simulink model "gm_smartCart3111"  (R2016a)
settings: Solver=FixedStepDiscrete  StartTime=0.0  StopTime=inf  FixedStep=1  RelTol=1e-3
libraries: simulink x92, hdlsllib x50
(part 1 of 3)
settings Model: Creator=Admin  LastModifiedBy=Admin
settings OptimizationCC: BlockReduction=off  ConditionallyExecuteInputs=off  DefaultParameterBehavior=Inlined
settings DebuggingCC: AlgebraicLoopMsg=error  InheritedTsInSrcMsg=none  MultiTaskCondExecSysMsg=warning  MultiTaskRateTransMsg=warning
settings HardwareCC: ProdBitPerPointer=32  ProdLargestAtomicFloat=None  ProdIntDivRoundTo=Undefined  ProdEndianess=Unspecified  ProdWordSize=32  ProdHWDeviceType=ASIC/FPGA->ASIC/FPGA  ProdEqTarget=off

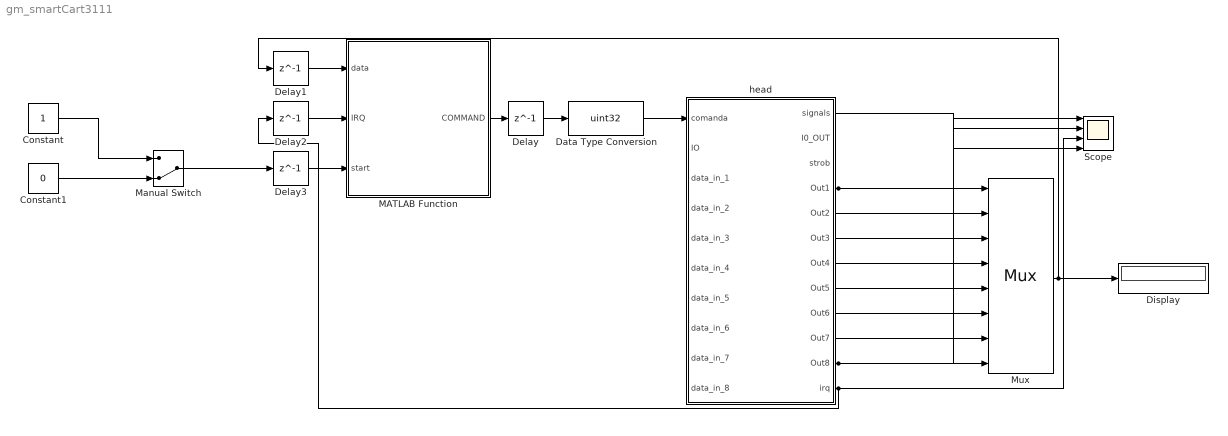
== system gm_smartCart3111 ==
  Constant : Constant  OutDataTypeStr=uint8
  Constant1 : Constant  Value=0  OutDataTypeStr=uint8
  Data Type Conversion : DataTypeConversion  OutDataTypeStr=uint32
  Delay{,1..3} (4 alike) : Delay  DelayLength=1  InitialCondition=0
  Display : Display
  MATLAB Function : MATLAB Function  TreatAsAtomicUnit=on
  Manual Switch : ManualSwitch  CurrentSetting=0
  Mux : Mux  Inputs=8
  Scope : Scope  NumInputPorts=4
  head : Subsystem  TreatAsAtomicUnit=on
  wires:
  Manual Switch/1 -> Delay3/1
  Delay3/1 -> MATLAB Function/3(start)
  Delay2/1 -> MATLAB Function/2(IRQ)
  Delay1/1 -> MATLAB Function/1(data)
  MATLAB Function/1(COMMAND) -> Delay/1
  Delay/1 -> Data Type Conversion/1
  head/1(signals) -> Scope/4
  head/11(Out8) -> Mux/8, Scope/2
  Data Type Conversion/1 -> head/1(comanda)
  Mux/1 -> Display/1, Delay1/1
  head/10(Out7) -> Mux/7
  head/9(Out6) -> Mux/6
  head/8(Out5) -> Mux/5
  head/7(Out4) -> Mux/4
  head/6(Out3) -> Mux/3
  head/5(Out2) -> Mux/2
  head/4(Out1) -> Mux/1, Scope/1
  head/12(irq) -> Scope/3, Delay2/1
  Constant1/1 -> Manual Switch/2
  Constant/1 -> Manual Switch/1

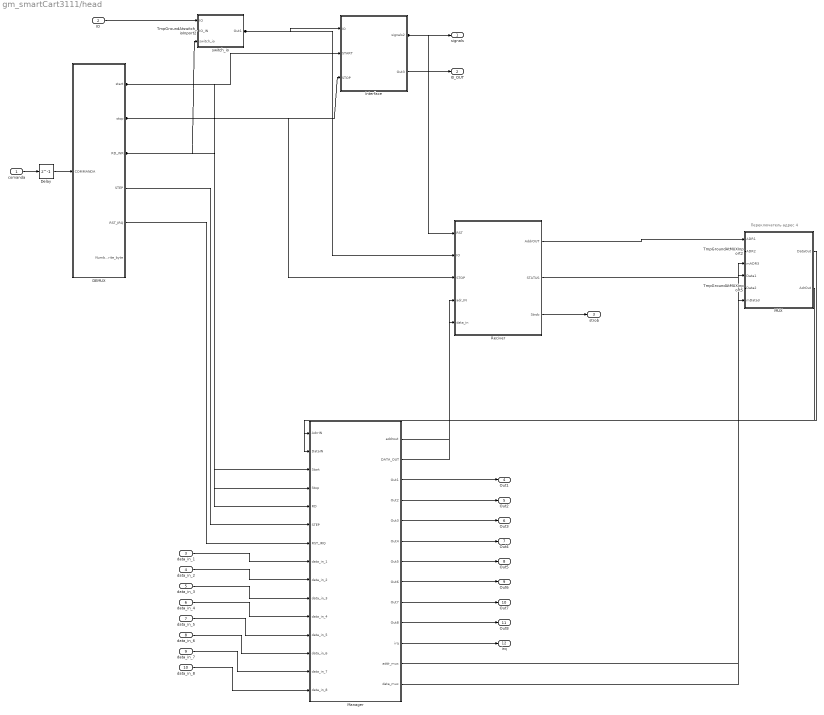
== system gm_smartCart3111/head ==
  note: Переключатель адрес 4
  comanda : Inport  OutDataTypeStr=uint32  SampleTime=1
  IO : Inport  Port=2  OutDataTypeStr=boolean
  data_in_1 : Inport  Port=3  OutDataTypeStr=uint32
  data_in_2 : Inport  Port=4  OutDataTypeStr=uint32
  data_in_3 : Inport  Port=5  OutDataTypeStr=uint32
  data_in_4 : Inport  Port=6  OutDataTypeStr=uint32
  data_in_5 : Inport  Port=7  OutDataTypeStr=uint32
  data_in_6 : Inport  Port=8  OutDataTypeStr=uint32
  data_in_7 : Inport  Port=9  OutDataTypeStr=uint32
  data_in_8 : Inport  Port=10  OutDataTypeStr=uint32
  DEMUX : Subsystem
  Delay : Delay  DelayLength=1  InitialCondition=0
  Interface : Subsystem
  MUX : Subsystem
  Manager : Subsystem
  Reciver : Subsystem
  TmpGroundAtMUXInport2 : Ground  DisableCoverage=on
  TmpGroundAtMUXInport5 : Ground  DisableCoverage=on
  TmpGroundAtswitch_ioInport2 : Ground  DisableCoverage=on
  switch_io : Subsystem
  signals : Outport  OutDataTypeStr=fixdt(1,4,0)
  I0_OUT : Outport  Port=2  OutDataTypeStr=boolean
  strob : Outport  Port=3  OutDataTypeStr=boolean
  Out1 : Outport  Port=4  OutDataTypeStr=uint8
  Out2 : Outport  Port=5  OutDataTypeStr=uint8
  Out3 : Outport  Port=6  OutDataTypeStr=uint8
  Out4 : Outport  Port=7  OutDataTypeStr=uint8
  Out5 : Outport  Port=8  OutDataTypeStr=uint8
  Out6 : Outport  Port=9  OutDataTypeStr=uint8
  Out7 : Outport  Port=10  OutDataTypeStr=uint8
  Out8 : Outport  Port=11  OutDataTypeStr=uint8
  irq : Outport  Port=12  OutDataTypeStr=boolean
  wires:
  comanda/1 -> Delay/1
  IO/1 -> switch_io/1(IO)
  data_in_1/1 -> Manager/8(data_in_1)
  data_in_2/1 -> Manager/9(data_in_2)
  data_in_3/1 -> Manager/10(data_in_3)
  data_in_4/1 -> Manager/11(data_in_4)
  data_in_5/1 -> Manager/12(data_in_5)
  data_in_6/1 -> Manager/13(data_in_6)
  data_in_7/1 -> Manager/14(data_in_7)
  data_in_8/1 -> Manager/15(data_in_8)
  DEMUX/1(start) -> Interface/2(START), Manager/3(Start)
  DEMUX/2(stop) -> Interface/3(STOP), Reciver/3(STOP), Manager/4(Stop)
  DEMUX/3(RD_WR) -> switch_io/3(switch_io), Manager/5(RD)
  DEMUX/4(STEP) -> Manager/6(STEP)
  DEMUX/5(RST_IRQ) -> Manager/7(RST_IRQ)
  Delay/1 -> DEMUX/1(COMMANDA)
  Interface/1(signals2) -> Reciver/1(RST), signals/1
  Interface/2(Out3) -> I0_OUT/1
  MUX/1(DataOut) -> Manager/2(DataIN)
  MUX/2(AdrOut) -> Manager/1(AdrrIN)
  Manager/1(addrout) -> Reciver/4(adr_IN)
  Manager/2(DATA_OUT) -> Reciver/5(data_in)
  Manager/3(Out1) -> Out1/1
  Manager/4(Out2) -> Out2/1
  Manager/5(Out3) -> Out3/1
  Manager/6(Out4) -> Out4/1
  Manager/7(Out5) -> Out5/1
  Manager/8(Out6) -> Out6/1
  Manager/9(Out7) -> Out7/1
  Manager/10(Out8) -> Out8/1
  Manager/11(irq) -> irq/1
  Manager/12(addr_mux) -> MUX/3(mADR3)
  Manager/13(data_mux) -> MUX/6(mData3)
  Reciver/1(AddrOUT) -> MUX/1(ADR1)
  Reciver/2(STATUS) -> MUX/4(Data1)
  Reciver/3(Strob) -> strob/1
  TmpGroundAtMUXInport2/1 -> MUX/2(ADR2)
  TmpGroundAtMUXInport5/1 -> MUX/5(Data2)
  TmpGroundAtswitch_ioInport2/1 -> switch_io/2(IO_IN)
  switch_io/1(Out1) -> Interface/1(IO), Reciver/2(IO)

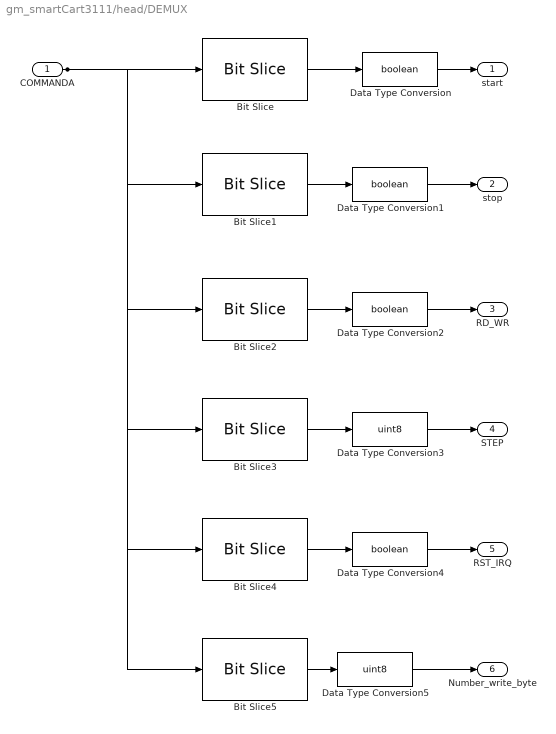
== system gm_smartCart3111/head/DEMUX ==
  COMMANDA : Inport  OutDataTypeStr=uint32  SampleTime=1
  Bit Slice : hdlsllib/HDL Operations/Bit Slice  lidx=0  ridx=0
  Bit Slice1 : hdlsllib/HDL Operations/Bit Slice  lidx=1  ridx=1
  Bit Slice2 : hdlsllib/HDL Operations/Bit Slice  lidx=2  ridx=2
  Bit Slice3 : hdlsllib/HDL Operations/Bit Slice  lidx=11  ridx=3
  Bit Slice4 : hdlsllib/HDL Operations/Bit Slice  lidx=12  ridx=12
  Bit Slice5 : hdlsllib/HDL Operations/Bit Slice  lidx=15  ridx=13
  Data Type Conversion{,1..2,4} (4 alike) : DataTypeConversion  OutDataTypeStr=boolean
  Data Type Conversion3 : DataTypeConversion  OutDataTypeStr=uint8
  Data Type Conversion5 : DataTypeConversion  OutDataTypeStr=uint8
  start : Outport
  stop : Outport  Port=2
  RD_WR : Outport  Port=3
  STEP : Outport  Port=4  OutDataTypeStr=uint8
  RST_IRQ : Outport  Port=5
  Number_write_byte : Outport  Port=6  OutDataTypeStr=uint8
  wires:
  COMMANDA/1 -> Bit Slice5/1, Bit Slice4/1, Bit Slice3/1, Bit Slice2/1, Bit Slice1/1, Bit Slice/1
  Bit Slice/1 -> Data Type Conversion/1
  Bit Slice1/1 -> Data Type Conversion1/1
  Bit Slice2/1 -> Data Type Conversion2/1
  Bit Slice3/1 -> Data Type Conversion3/1
  Bit Slice4/1 -> Data Type Conversion4/1
  Bit Slice5/1 -> Data Type Conversion5/1
  Data Type Conversion/1 -> start/1
  Data Type Conversion1/1 -> stop/1
  Data Type Conversion2/1 -> RD_WR/1
  Data Type Conversion3/1 -> STEP/1
  Data Type Conversion4/1 -> RST_IRQ/1
  Data Type Conversion5/1 -> Number_write_byte/1

== system gm_smartCart3111/head/Interface ==
  IO : Inport  OutDataTypeStr=boolean
  START : Inport  Port=2  OutDataTypeStr=boolean  SampleTime=1
  STOP : Inport  Port=3  OutDataTypeStr=boolean  SampleTime=1
  ColdStart : Subsystem
  ColdStop2 : Subsystem
  Head2 : Subsystem
  MUX2 : Subsystem
  Swith_signal2 : Subsystem
  signals2 : Outport  OutDataTypeStr=fixdt(1,4,0)  InitialOutput=0
  Out3 : Outport  Port=2  OutDataTypeStr=boolean  InitialOutput=0
  wires:
  IO/1 -> Out3/1, ColdStart/1(Reqest)
  START/1 -> Head2/3(START)
  STOP/1 -> Head2/4(STOP)
  ColdStart/1(DataOUT) -> MUX2/5(DAT_ST1)
  ColdStart/2(Signal) -> MUX2/2(DATA_0)
  ColdStart/3(ADR_OUT) -> MUX2/4(ADR_ST)
  ColdStop2/1(DataOUT) -> MUX2/7(DAT_STOP)
  ColdStop2/2(Signal) -> MUX2/3(DATA_1)
  ColdStop2/3(ADR_OUT) -> MUX2/6(ADR_STOP)
  Head2/1(AdrOut) -> Swith_signal2/1(Adr), ColdStart/2(Addr), ColdStop2/1(Addr)
  Head2/2(DataOut) -> Swith_signal2/2(Data), ColdStart/3(Data), ColdStop2/2(Data)
  MUX2/1(Signals) -> signals2/1
  MUX2/2(ADR_OUT) -> Head2/1(ADR_IN)
  MUX2/3(DATA_OUT1) -> Head2/2(DataIN)
  Swith_signal2/1(OutAddr) -> MUX2/1(ADR)

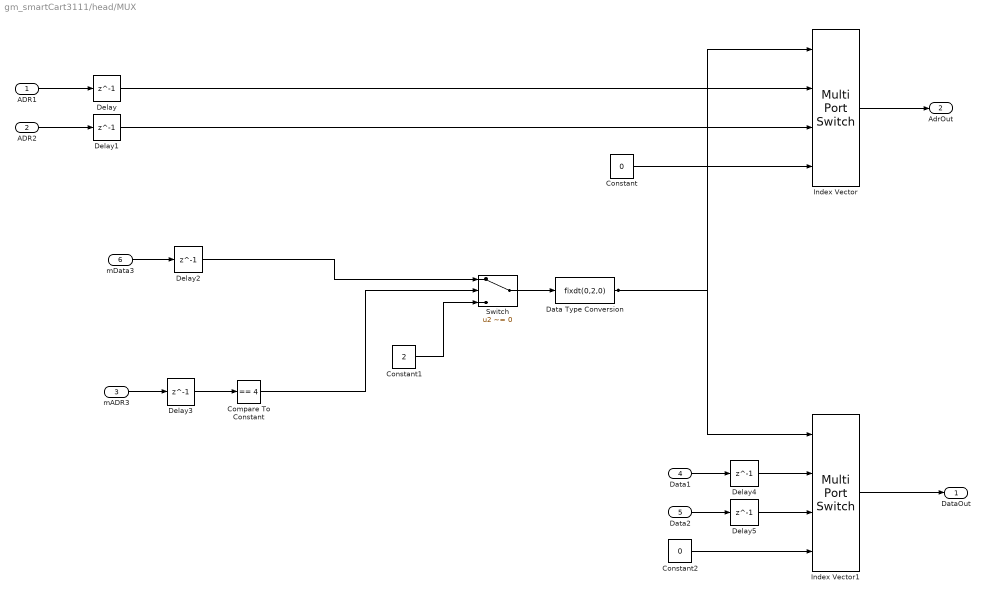
== system gm_smartCart3111/head/MUX ==
  ADR1 : Inport  OutDataTypeStr=uint8  SampleTime=1
  ADR2 : Inport  Port=2  OutDataTypeStr=uint8
  mADR3 : Inport  Port=3  OutDataTypeStr=uint8  SampleTime=1
  Data1 : Inport  Port=4  OutDataTypeStr=uint32  SampleTime=1
  Data2 : Inport  Port=5  OutDataTypeStr=uint32
  mData3 : Inport  Port=6  OutDataTypeStr=uint32  SampleTime=1
  Compare To Constant : simulink/Logic and Bit Operations/Compare To Constant  relop===  const=4  OutDataTypeStr=boolean
  Constant : Constant  Value=0  OutDataTypeStr=uint8
  Constant1 : Constant  Value=2  OutDataTypeStr=uint32
  Constant2 : Constant  Value=0  OutDataTypeStr=uint32
  Data Type Conversion : DataTypeConversion  OutDataTypeStr=fixdt(0,2,0)
  Delay{,1..5} (6 alike) : Delay  DelayLength=1  InitialCondition=0
  Index Vector : MultiPortSwitch  DataPortOrder=Zero-based contiguous  zeroidx=on
  Index Vector1 : MultiPortSwitch  DataPortOrder=Zero-based contiguous  zeroidx=on
  Switch : Switch  Criteria=u2 ~= 0
  DataOut : Outport  OutDataTypeStr=uint32
  AdrOut : Outport  Port=2  OutDataTypeStr=uint8
  wires:
  ADR1/1 -> Delay/1
  ADR2/1 -> Delay1/1
  mADR3/1 -> Delay3/1
  Data1/1 -> Delay4/1
  Data2/1 -> Delay5/1
  mData3/1 -> Delay2/1
  Compare To Constant/1 -> Switch/2
  Constant/1 -> Index Vector/4
  Constant1/1 -> Switch/3
  Constant2/1 -> Index Vector1/4
  Data Type Conversion/1 -> Index Vector1/1, Index Vector/1
  Delay/1 -> Index Vector/2
  Delay1/1 -> Index Vector/3
  Delay2/1 -> Switch/1
  Delay3/1 -> Compare To Constant/1
  Delay4/1 -> Index Vector1/2
  Delay5/1 -> Index Vector1/3
  Index Vector/1 -> AdrOut/1
  Index Vector1/1 -> DataOut/1
  Switch/1 -> Data Type Conversion/1

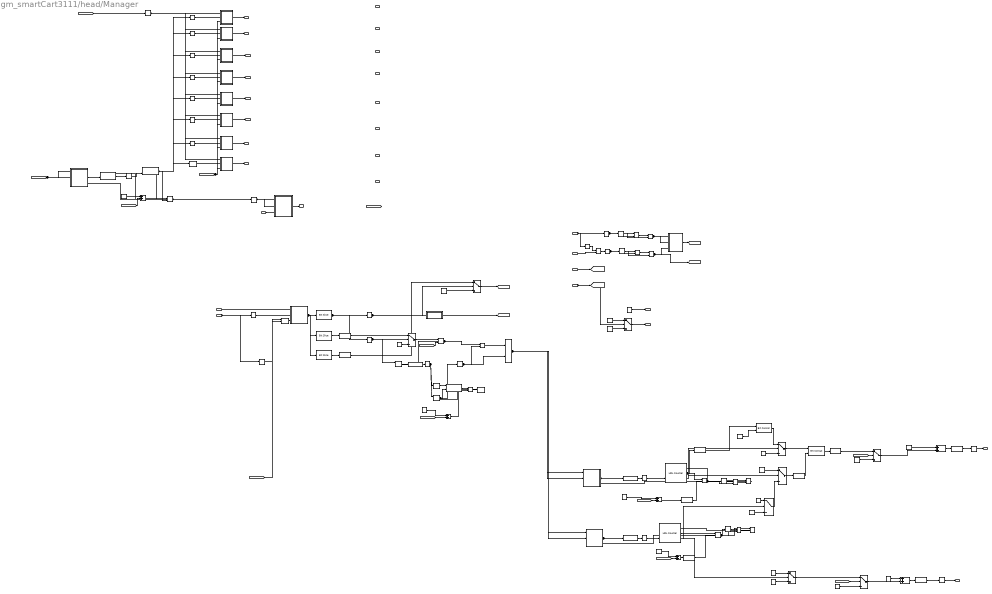
== system gm_smartCart3111/head/Manager ==
  note: Схема управления приёмника
  note: Схема включения и выключения
  note: Схема синхр
  note: Схема декодирования команд
  note: Декодер команд
  AdrrIN : Inport  OutDataTypeStr=uint8  SampleTime=1
  DataIN : Inport  Port=2  OutDataTypeStr=uint32  SampleTime=1
  Start : Inport  Port=3  OutDataTypeStr=boolean  SampleTime=1
  Stop : Inport  Port=4  OutDataTypeStr=boolean  SampleTime=1
  RD : Inport  Port=5  OutDataTypeStr=boolean  SampleTime=1
  STEP : Inport  Port=6  OutDataTypeStr=uint8  SampleTime=1
  RST_IRQ : Inport  Port=7  OutDataTypeStr=boolean  SampleTime=1
  data_in_1 : Inport  Port=8  OutDataTypeStr=uint32
  data_in_2 : Inport  Port=9  OutDataTypeStr=uint32
  data_in_3 : Inport  Port=10  OutDataTypeStr=uint32
  data_in_4 : Inport  Port=11  OutDataTypeStr=uint32
  data_in_5 : Inport  Port=12  OutDataTypeStr=uint32
  data_in_6 : Inport  Port=13  OutDataTypeStr=uint32
  data_in_7 : Inport  Port=14  OutDataTypeStr=uint32
  data_in_8 : Inport  Port=15  OutDataTypeStr=uint32
  Add{,1..5} (6 alike) : Sum
  Bit Concat : hdlsllib/HDL Operations/Bit Concat  numInputs=2
  Bit Concat1 : hdlsllib/HDL Operations/Bit Concat  numInputs=2
  Bit Slice3 : hdlsllib/HDL Operations/Bit Slice  lidx=1  ridx=0
  Bit Slice4 : hdlsllib/HDL Operations/Bit Slice  lidx=9  ridx=2
  Bit Slice5 : hdlsllib/HDL Operations/Bit Slice  lidx=17  ridx=10
  Compare To Constant{,1..6,10,12} (9 alike) : simulink/Logic and Bit Operations/Compare To Constant  relop===  const=1  OutDataTypeStr=boolean
  Compare To Constant11 : simulink/Logic and Bit Operations/Compare To Constant  relop===  const=4  OutDataTypeStr=boolean
  Compare To Constant13 : simulink/Logic and Bit Operations/Compare To Constant  relop===  const=2  OutDataTypeStr=boolean
  Compare To Constant14 : simulink/Logic and Bit Operations/Compare To Constant  relop===  const=5  OutDataTypeStr=boolean
  Compare To Constant15 : simulink/Logic and Bit Operations/Compare To Constant  relop===  const=6  OutDataTypeStr=boolean
  Compare To Constant16 : simulink/Logic and Bit Operations/Compare To Constant  relop===  const=7  OutDataTypeStr=boolean
  Compare To Constant17 : simulink/Logic and Bit Operations/Compare To Constant  relop===  const=8  OutDataTypeStr=boolean
  Compare To Constant7 : simulink/Logic and Bit Operations/Compare To Constant  relop===  const=2  OutDataTypeStr=boolean
  Compare To Constant8 : simulink/Logic and Bit Operations/Compare To Constant  relop===  const=3  OutDataTypeStr=boolean
  Compare To Constant9 : simulink/Logic and Bit Operations/Compare To Constant  relop===  const=2  OutDataTypeStr=boolean
  Constant{,2,14..15,23,25,29..30} (8 alike) : Constant  Value=0  OutDataTypeStr=uint8  SampleTime=-1
  Constant{1,3,7,10,24} (5 alike) : Constant  OutDataTypeStr=uint8  SampleTime=-1
  Constant11 : Constant  Value=4  OutDataTypeStr=uint8  SampleTime=-1
  Constant22 : Constant  Value=0  OutDataTypeStr=uint32  SampleTime=-1
  Constant4 : Constant  Value=2  OutDataTypeStr=uint8  SampleTime=-1
  Constant5 : Constant  OutDataTypeStr=boolean  SampleTime=-1
  Constant6 : Constant  Value=0  OutDataTypeStr=uint32  SampleTime=-1
  Constant8 : Constant  OutDataTypeStr=uint32  SampleTime=-1
  Constant9 : Constant  Value=2  OutDataTypeStr=uint8  SampleTime=-1
  Data Type Conversion{,4,7..8} (4 alike) : DataTypeConversion  OutDataTypeStr=uint8
  Data Type Conversion1 : DataTypeConversion  OutDataTypeStr=uint32
  Data Type Conversion10 : DataTypeConversion  OutDataTypeStr=fixdt(0,2,0)
  Data Type Conversion5 : DataTypeConversion  OutDataTypeStr=uint32
  Data Type Conversion6 : DataTypeConversion  OutDataTypeStr=fixdt(0,4,0)
  Data Type Conversion9 : DataTypeConversion  OutDataTypeStr=fixdt(0,4,0)
  Delay{,1..3,5..8} (8 alike) : Delay  DelayLength=1  InitialCondition=0
  Delay4 : Delay  DelayLength=3  InitialCondition=0
  HDL Counter1 : hdlsllib/HDL Operations/HDL Counter  CountType=Free running  CountInit=0  CountStep=1  CountMax=25  CountFromType=Initial value  CountFrom=0  CountResetPort=on  CountLoadPort=off  CountEnbPort=on  CountDirPort=off  CountDataType=Unsigned  CountWordLen=4  CountFracLen=0  CountSampTime=1
  HDL Counter2 : hdlsllib/HDL Operations/HDL Counter  CountType=Free running  CountInit=0  CountStep=1  CountMax=25  CountFromType=Initial value  CountFrom=0  CountResetPort=on  CountLoadPort=off  CountEnbPort=on  CountDirPort=off  CountDataType=Unsigned  CountWordLen=4  CountFracLen=0  CountSampTime=1
  HDL Counter3 : hdlsllib/HDL Operations/HDL Counter  CountType=Free running  CountInit=0  CountStep=1  CountMax=25  CountFromType=Initial value  CountFrom=0  CountResetPort=on  CountLoadPort=off  CountEnbPort=on  CountDirPort=off  CountDataType=Unsigned  CountWordLen=8  CountFracLen=0  CountSampTime=1
  HDL Counter4 : hdlsllib/HDL Operations/HDL Counter  CountType=Free running  CountInit=0  CountStep=1  CountMax=25  CountFromType=Initial value  CountFrom=0  CountResetPort=on  CountLoadPort=off  CountEnbPort=on  CountDirPort=off  CountDataType=Unsigned  CountWordLen=4  CountFracLen=0  CountSampTime=1
  HDL Counter5 : hdlsllib/HDL Operations/HDL Counter  CountType=Free running  CountInit=0  CountStep=1  CountMax=25  CountFromType=Initial value  CountFrom=0  CountResetPort=off  CountLoadPort=off  CountEnbPort=on  CountDirPort=off  CountDataType=Unsigned  CountWordLen=1  CountFracLen=0  CountSampTime=1
  HDL Counter6 : hdlsllib/HDL Operations/HDL Counter  CountType=Free running  CountInit=0  CountStep=1  CountMax=25  CountFromType=Initial value  CountFrom=0  CountResetPort=off  CountLoadPort=off  CountEnbPort=on  CountDirPort=off  CountDataType=Unsigned  CountWordLen=1  CountFracLen=0  CountSampTime=1
  HDL Counter7 : hdlsllib/HDL Operations/HDL Counter  CountType=Free running  CountInit=0  CountStep=1  CountMax=25  CountFromType=Initial value  CountFrom=0  CountResetPort=off  CountLoadPort=off  CountEnbPort=on  CountDirPort=off  CountDataType=Unsigned  CountWordLen=1  CountFracLen=0  CountSampTime=1
  HDL Counter8 : hdlsllib/HDL Operations/HDL Counter  CountType=Free running  CountInit=0  CountStep=1  CountMax=25  CountFromType=Initial value  CountFrom=0  CountResetPort=on  CountLoadPort=off  CountEnbPort=on  CountDirPort=off  CountDataType=Unsigned  CountWordLen=1  CountFracLen=0  CountSampTime=1
  Logical Operator{,2,7,10} (4 alike) : Logic  Operator=XOR  AllPortsSameDT=off  OutDataTypeStr=boolean
  Logical Operator{1,3..4,6,8..9,12,17,19} (9 alike) : Logic  AllPortsSameDT=off  OutDataTypeStr=boolean
  Logical Operator11 : Logic  Operator=NOT  AllPortsSameDT=off  OutDataTypeStr=boolean
  Logical Operator14 : Logic  Operator=OR  AllPortsSameDT=off  OutDataTypeStr=boolean
  Logical Operator18 : Logic  Operator=NOT  AllPortsSameDT=off  OutDataTypeStr=boolean
  Logical Operator5 : Logic  Operator=NOT  AllPortsSameDT=off  OutDataTypeStr=boolean
  Relational Operator{,1..4} (5 alike) : RelationalOperator  Operator===  OutDataTypeStr=boolean
  Switch{1..3,5,9..10,12..14} (9 alike) : Switch  Criteria=u2 ~= 0
  Unit Delay Enabled Resettable : Subsystem
  Unit Delay Enabled Resettable1 : Subsystem
  Unit Delay Enabled Resettable10 : Subsystem
  Unit Delay Enabled Resettable11 : Subsystem
  Unit Delay Enabled Resettable12 : Subsystem
  Unit Delay Enabled Resettable13 : Subsystem
  Unit Delay Enabled Resettable14 : Subsystem
  Unit Delay Enabled Resettable3 : Subsystem
  Unit Delay Enabled Resettable4 : Subsystem
  Unit Delay Enabled Resettable5 : Subsystem
  Unit Delay Enabled Resettable6 : Subsystem
  Unit Delay Enabled Resettable7 : Subsystem
  Unit Delay Enabled Resettable8 : Subsystem
  Unit Delay Enabled Resettable9 : Subsystem
  signal_edg : Subsystem
  addrout : Outport  OutDataTypeStr=uint8
  DATA_OUT : Outport  Port=2  OutDataTypeStr=uint32
  Out1 : Outport  Port=3  OutDataTypeStr=uint8
  Out2 : Outport  Port=4  OutDataTypeStr=uint8
  Out3 : Outport  Port=5  OutDataTypeStr=uint8
  Out4 : Outport  Port=6  OutDataTypeStr=uint8
  Out5 : Outport  Port=7  OutDataTypeStr=uint8
  Out6 : Outport  Port=8  OutDataTypeStr=uint8
  Out7 : Outport  Port=9  OutDataTypeStr=uint8
  Out8 : Outport  Port=10  OutDataTypeStr=uint8
  irq : Outport  Port=11  OutDataTypeStr=boolean
  addr_mux : Outport  Port=12  OutDataTypeStr=uint8
  data_mux : Outport  Port=13  OutDataTypeStr=uint32
  wires:
  AdrrIN/1 -> Compare To Constant13/1, Compare To Constant12/1
  DataIN/1 -> Unit Delay Enabled Resettable1/1(data_in)
  Start/1 -> Logical Operator5/1, Compare To Constant/1
  Stop/1 -> Logical Operator4/2
  RD/1 -> Switch5/2, [INST_WORK]
  STEP/1 -> [INST_WORK_VAL]
  RST_IRQ/1 -> Unit Delay Enabled Resettable14/3(Reset)
  Add/1 -> Data Type Conversion6/1
  Add1/1 -> Data Type Conversion4/1
  Add2/1 -> Data Type Conversion5/1
  Add3/1 -> Data Type Conversion9/1
  Add4/1 -> Relational Operator3/1
  Add5/1 -> Relational Operator4/2
  Bit Concat/1 -> Data Type Conversion1/1
  Bit Concat1/1 -> Switch2/1
  Bit Slice3/1 -> Compare To Constant9/1, Compare To Constant10/1
  Bit Slice4/1 -> Data Type Conversion7/1
  Bit Slice5/1 -> Data Type Conversion8/1
  Compare To Constant/1 -> Logical Operator1/2, Logical Operator/2, Delay/1
  Compare To Constant1/1 -> Logical Operator3/2, Logical Operator2/2, Delay1/1
  Compare To Constant10/1 -> Switch10/2, Logical Operator19/1
  Compare To Constant11/1 -> Unit Delay Enabled Resettable9/2(Enb)
  Compare To Constant12/1 -> Unit Delay Enabled Resettable1/2(Enb)
  Compare To Constant13/1 -> Logical Operator14/2
  Compare To Constant14/1 -> Unit Delay Enabled Resettable10/2(Enb)
  Compare To Constant15/1 -> Unit Delay Enabled Resettable11/2(Enb)
  Compare To Constant16/1 -> Unit Delay Enabled Resettable12/2(Enb)
  Compare To Constant17/1 -> Unit Delay Enabled Resettable13/2(Enb)
  Compare To Constant2/1 -> HDL Counter3/2
  Compare To Constant3/1 -> Logical Operator12/1, Logical Operator11/1
  Compare To Constant4/1 -> HDL Counter1/2
  Compare To Constant5/1 -> HDL Counter2/2
  Compare To Constant6/1 -> Unit Delay Enabled Resettable6/2(Enb)
  Compare To Constant7/1 -> Unit Delay Enabled Resettable7/2(Enb)
  Compare To Constant8/1 -> Unit Delay Enabled Resettable8/2(Enb)
  Compare To Constant9/1 -> Switch9/2, signal_edg/1(In1)
  Constant/1 -> Switch2/3
  Constant1/1 -> Switch1/1
  Constant10/1 -> Add5/1
  Constant11/1 -> addr_mux/1
  Constant14/1 -> Switch9/3
  Constant15/1 -> Switch10/3
  Constant2/1 -> Switch1/3
  Constant22/1 -> Switch12/3
  Constant23/1 -> Switch13/3
  Constant24/1 -> Add3/1
  Constant25/1 -> Switch14/3
  Constant29/1 -> Add1/1
  Constant3/1 -> Switch14/1
  Constant30/1 -> Add2/1
  Constant4/1 -> Switch3/1
  Constant5/1 -> Bit Concat1/2
  Constant6/1 -> Switch5/1
  Constant7/1 -> Add4/1
  Constant8/1 -> Switch5/3
  Constant9/1 -> Add/1
  Data Type Conversion/1 -> Bit Concat1/1
  Data Type Conversion1/1 -> Switch12/1
  Data Type Conversion10/1 -> Bit Concat/2
  Data Type Conversion4/1 -> Delay8/1
  Data Type Conversion5/1 -> Delay7/1
  Data Type Conversion6/1 -> Relational Operator2/2
  Data Type Conversion7/1 -> Switch10/1
  Data Type Conversion8/1 -> Switch9/1
  Data Type Conversion9/1 -> Relational Operator1/2
  Delay/1 -> Logical Operator/1
  Delay1/1 -> Logical Operator2/1
  Delay2/1 -> Logical Operator7/1
  Delay3/1 -> Logical Operator10/1
  Delay4/1 -> Unit Delay Enabled Resettable9/1(data_in), Unit Delay Enabled Resettable8/1(data_in), Unit Delay Enabled Resettable7/1(data_in), Unit Delay Enabled Resettable6/1(data_in), Unit Delay Enabled Resettable13/1(data_in), Unit Delay Enabled Resettable12/1(data_in), Unit Delay Enabled Resettable11/1(data_in), Unit Delay Enabled Resettable10/1(data_in)
  Delay5/1 -> Unit Delay Enabled Resettable14/2(Enb), Unit Delay Enabled Resettable14/1(data_in)
  Delay6/1 -> Logical Operator8/2, Logical Operator17/2
  Delay7/1 -> DATA_OUT/1
  Delay8/1 -> addrout/1
  [INST_WORK_VAL] -> Relational Operator/2
  [INST_WORK_VAL] -> Add5/2
  [RST] -> Unit Delay Enabled Resettable9/3(Reset), Unit Delay Enabled Resettable8/3(Reset), Unit Delay Enabled Resettable7/3(Reset), Unit Delay Enabled Resettable6/3(Reset), Unit Delay Enabled Resettable13/3(Reset), Unit Delay Enabled Resettable12/3(Reset), Unit Delay Enabled Resettable11/3(Reset), Unit Delay Enabled Resettable10/3(Reset)
  [INST_WORK_VAL] -> Add/2
  [RST] -> Logical Operator14/1
  [RD_BYTE] -> Unit Delay Enabled Resettable5/2(Enb), Unit Delay Enabled Resettable5/1(data_in)
  [INST_WORK] -> Switch12/2
  [INST_WORK] -> Switch13/2
  [INST_WORK_VAL] -> Add3/2
  [RD_BYTE_VAL] -> Delay4/1
  [INST_WORK_VAL] -> Add4/2
  HDL Counter1/1 -> Relational Operator1/1, Data Type Conversion/1
  HDL Counter2/1 -> Relational Operator2/1
  HDL Counter3/1 -> Relational Operator3/2, Compare To Constant8/1, Compare To Constant7/1, Compare To Constant6/1, Compare To Constant17/1, Compare To Constant16/1, Compare To Constant15/1, Compare To Constant14/1, Compare To Constant11/1
  HDL Counter4/1 -> Relational Operator4/1
  HDL Counter5/1 -> Compare To Constant3/1
  HDL Counter6/1 -> Compare To Constant4/1
  HDL Counter7/1 -> Compare To Constant5/1
  HDL Counter8/1 -> Compare To Constant2/1
  Logical Operator/1 -> Logical Operator1/1
  Logical Operator1/1 -> Unit Delay Enabled Resettable/2(Enb), Unit Delay Enabled Resettable/1(data_in)
  Logical Operator10/1 -> Logical Operator9/2
  Logical Operator11/1 -> HDL Counter4/1
  Logical Operator12/1 -> HDL Counter4/2, Delay6/1
  Logical Operator14/1 -> Unit Delay Enabled Resettable1/3(Reset)
  Logical Operator17/1 -> Logical Operator8/1
  Logical Operator18/1 -> Logical Operator12/2
  Logical Operator19/1 -> HDL Counter5/1
  Logical Operator2/1 -> Logical Operator3/1
  Logical Operator3/1 -> Unit Delay Enabled Resettable/3(Reset), [RST]
  Logical Operator4/1 -> Compare To Constant1/1
  Logical Operator5/1 -> Logical Operator4/1
  Logical Operator6/1 -> HDL Counter1/1
  Logical Operator7/1 -> Logical Operator6/2
  Logical Operator8/1 -> Unit Delay Enabled Resettable4/2(Enb), Unit Delay Enabled Resettable4/1(data_in), Unit Delay Enabled Resettable3/2(Enb), Unit Delay Enabled Resettable3/1(data_in)
  Logical Operator9/1 -> HDL Counter2/1
  Relational Operator/1 -> Logical Operator19/2, Logical Operator17/1
  Relational Operator1/1 -> Logical Operator7/2, Logical Operator6/1, Unit Delay Enabled Resettable3/3(Reset), Delay2/1
  Relational Operator2/1 -> Logical Operator9/1, Logical Operator10/2, Unit Delay Enabled Resettable4/3(Reset), Delay3/1
  Relational Operator3/1 -> Unit Delay Enabled Resettable5/3(Reset), HDL Counter8/1, HDL Counter3/1, Delay5/1
  Relational Operator4/1 -> Logical Operator18/1
  Switch1/1 -> Switch13/1
  Switch10/1 -> Relational Operator/1
  Switch12/1 -> Add2/2
  Switch13/1 -> Add1/2
  Switch14/1 -> Switch3/3
  Switch2/1 -> Bit Concat/1
  Switch3/1 -> Data Type Conversion10/1
  Switch5/1 -> data_mux/1
  Switch9/1 -> [RD_BYTE_VAL]
  Unit Delay Enabled Resettable/1(data_out) -> [EN]
  Unit Delay Enabled Resettable1/1(data_out) -> Bit Slice5/1, Bit Slice4/1, Bit Slice3/1
  Unit Delay Enabled Resettable10/1(data_out) -> Out5/1
  Unit Delay Enabled Resettable11/1(data_out) -> Out6/1
  Unit Delay Enabled Resettable12/1(data_out) -> Out7/1
  Unit Delay Enabled Resettable13/1(data_out) -> Out8/1
  Unit Delay Enabled Resettable14/1(data_out) -> irq/1
  Unit Delay Enabled Resettable3/1(data_out) -> Switch3/2, Switch2/2, HDL Counter6/1
  Unit Delay Enabled Resettable4/1(data_out) -> Switch14/2, Switch1/2, HDL Counter7/1
  Unit Delay Enabled Resettable5/1(data_out) -> HDL Counter8/2
  Unit Delay Enabled Resettable6/1(data_out) -> Out1/1
  Unit Delay Enabled Resettable7/1(data_out) -> Out2/1
  Unit Delay Enabled Resettable8/1(data_out) -> Out3/1
  Unit Delay Enabled Resettable9/1(data_out) -> Out4/1
  signal_edg/1(Out1) -> [RD_BYTE]

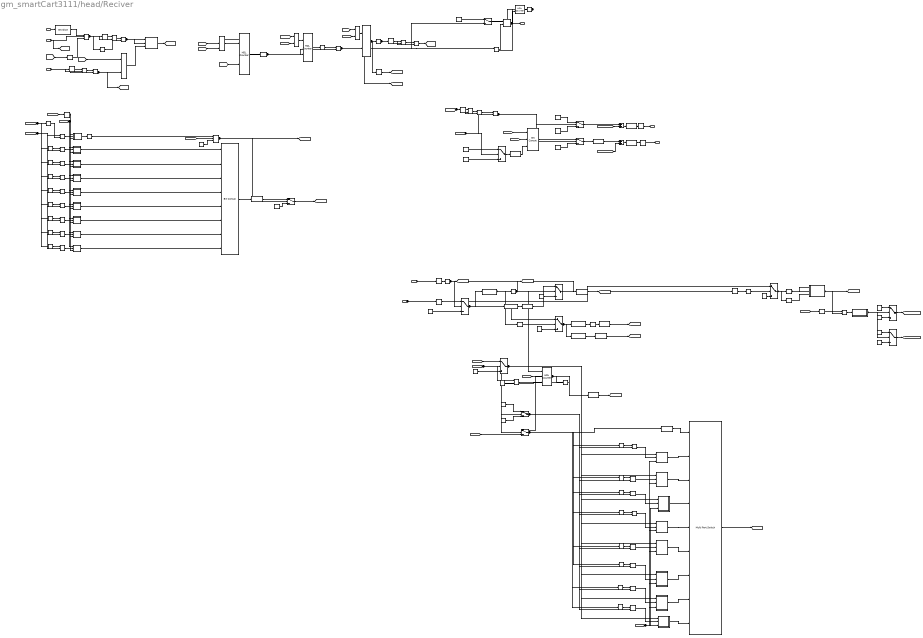
== system gm_smartCart3111/head/Reciver ==
  note: Схема обнаружение сообщения (1)
  note: cхема управления и синхронизации (2)
  note: Схема формирования отчёта о работе приёмника (4)
  note: Схема связи (5)
  note: Cхема формирования байта и проверка четности
  RST : Inport  OutDataTypeStr=fixdt(1,4,0)  SampleTime=1
  IO : Inport  Port=2  OutDataTypeStr=boolean
  STOP : Inport  Port=3  OutDataTypeStr=boolean  SampleTime=1
  adr_IN : Inport  Port=4  OutDataTypeStr=uint8  SampleTime=1
  data_in : Inport  Port=5  OutDataTypeStr=uint32  SampleTime=1
  Add : Sum
  Add1 : Sum
  Bit Concat : hdlsllib/HDL Operations/Bit Concat  numInputs=8
  Bit Concat1 : hdlsllib/HDL Operations/Bit Concat  numInputs=3
  Bit Slice1 : hdlsllib/HDL Operations/Bit Slice  lidx=3  ridx=3
  Bit Slice2 : hdlsllib/HDL Operations/Bit Slice  lidx=1  ridx=0
  Bit Slice3 : hdlsllib/HDL Operations/Bit Slice  lidx=7  ridx=2
  Bit Slice4 : hdlsllib/HDL Operations/Bit Slice  lidx=2  ridx=2
  Bit Slice5 : hdlsllib/HDL Operations/Bit Slice  lidx=8  ridx=3
  Compare To Constant{1,3,13,21,31..32} (6 alike) : simulink/Logic and Bit Operations/Compare To Constant  relop===  const=0  OutDataTypeStr=boolean
  Compare To Constant10 : simulink/Logic and Bit Operations/Compare To Constant  relop===  const=7  OutDataTypeStr=boolean
  Compare To Constant11 : simulink/Logic and Bit Operations/Compare To Constant  relop===  const=8  OutDataTypeStr=boolean
  Compare To Constant14 : simulink/Logic and Bit Operations/Compare To Constant  relop===  const=6  OutDataTypeStr=boolean
  Compare To Constant15 : simulink/Logic and Bit Operations/Compare To Constant  relop===  const=7  OutDataTypeStr=boolean
  Compare To Constant{5,16,18,20,22,30} (6 alike) : simulink/Logic and Bit Operations/Compare To Constant  relop===  const=1  OutDataTypeStr=boolean
  Compare To Constant17 : simulink/Logic and Bit Operations/Compare To Constant  relop===  const=200  OutDataTypeStr=boolean
  Compare To Constant19 : simulink/Logic and Bit Operations/Compare To Constant  relop===  const=2  OutDataTypeStr=boolean
  Compare To Constant2 : simulink/Logic and Bit Operations/Compare To Constant  relop===  const=10  OutDataTypeStr=boolean
  Compare To Constant23 : simulink/Logic and Bit Operations/Compare To Constant  relop===  const=2  OutDataTypeStr=boolean
  Compare To Constant24 : simulink/Logic and Bit Operations/Compare To Constant  relop===  const=3  OutDataTypeStr=boolean
  Compare To Constant25 : simulink/Logic and Bit Operations/Compare To Constant  relop===  const=4  OutDataTypeStr=boolean
  Compare To Constant26 : simulink/Logic and Bit Operations/Compare To Constant  relop===  const=5  OutDataTypeStr=boolean
  Compare To Constant27 : simulink/Logic and Bit Operations/Compare To Constant  relop===  const=6  OutDataTypeStr=boolean
  Compare To Constant28 : simulink/Logic and Bit Operations/Compare To Constant  relop===  const=7  OutDataTypeStr=boolean
  Compare To Constant29 : simulink/Logic and Bit Operations/Compare To Constant  relop===  const=5  OutDataTypeStr=boolean
  Compare To Constant4 : simulink/Logic and Bit Operations/Compare To Constant  relop===  const=2604  OutDataTypeStr=boolean
  Compare To Constant6 : simulink/Logic and Bit Operations/Compare To Constant  relop===  const=2  OutDataTypeStr=boolean
  Compare To Constant7 : simulink/Logic and Bit Operations/Compare To Constant  relop===  const=3  OutDataTypeStr=boolean
  Compare To Constant8 : simulink/Logic and Bit Operations/Compare To Constant  relop===  const=4  OutDataTypeStr=boolean
  Compare To Constant9 : simulink/Logic and Bit Operations/Compare To Constant  relop===  const=5  OutDataTypeStr=boolean
  Constant : Constant  Value=0  OutDataTypeStr=uint8
  Constant1 : Constant  Value=0  OutDataTypeStr=uint8
  Constant10 : Constant  Value=0  OutDataTypeStr=boolean  SampleTime=-1
  Constant11 : Constant  Value=0  OutDataTypeStr=boolean
  Constant12 : Constant  Value=0  OutDataTypeStr=uint8
  Constant{3,7,13..15} (5 alike) : Constant  Value=0  OutDataTypeStr=uint32  SampleTime=-1
  Constant16 : Constant  Value=0  OutDataTypeStr=uint8  SampleTime=-1
  Constant17 : Constant  Value=5  OutDataTypeStr=uint8  SampleTime=-1
  Constant18 : Constant  OutDataTypeStr=uint8  SampleTime=-1
  Constant2 : Constant  OutDataTypeStr=uint8
  Constant4 : Constant  Value=2  OutDataTypeStr=fixdt(0,2,0)
  Constant5 : Constant  Value=0  OutDataTypeStr=uint8  SampleTime=-1
  Constant6 : Constant  OutDataTypeStr=boolean
  Constant8 : Constant  OutDataTypeStr=fixdt(0,2,0)
  Constant9 : Constant  OutDataTypeStr=boolean
  Data Type Conversion : DataTypeConversion  OutDataTypeStr=uint8
  Data Type Conversion1 : DataTypeConversion  OutDataTypeStr=fixdt(0,5,0)
  Data Type Conversion10 : DataTypeConversion  OutDataTypeStr=uint8
  Data Type Conversion2 : DataTypeConversion  OutDataTypeStr=uint8
  Data Type Conversion3 : DataTypeConversion  OutDataTypeStr=boolean
  Data Type Conversion4 : DataTypeConversion  OutDataTypeStr=uint32
  Data Type Conversion5 : DataTypeConversion  OutDataTypeStr=uint32
  Data Type Conversion6 : DataTypeConversion  OutDataTypeStr=fixdt(0,5,0)
  Data Type Conversion7 : DataTypeConversion  OutDataTypeStr=fixdt(0,2,0)
  Data Type Conversion8 : DataTypeConversion  OutDataTypeStr=fixdt(1,4,0)
  Data Type Conversion9 : DataTypeConversion  OutDataTypeStr=uint32
  Delay{,1..9,11} (11 alike) : Delay  DelayLength=1  InitialCondition=0
  HDL Counter : hdlsllib/HDL Operations/HDL Counter  CountType=Free running  CountInit=0  CountStep=1  CountMax=1  CountFromType=Initial value  CountFrom=0  CountResetPort=on  CountLoadPort=off  CountEnbPort=on  CountDirPort=off  CountDataType=Unsigned  CountWordLen=13  CountFracLen=0  CountSampTime=1
  HDL Counter1 : hdlsllib/HDL Operations/HDL Counter  CountType=Free running  CountInit=0  CountStep=1  CountMax=1  CountFromType=Initial value  CountFrom=0  CountResetPort=on  CountLoadPort=off  CountEnbPort=on  CountDirPort=off  CountDataType=Unsigned  CountWordLen=1  CountFracLen=0  CountSampTime=1
  HDL Counter2 : hdlsllib/HDL Operations/HDL Counter  CountType=Count limited  CountInit=0  CountStep=1  CountMax=10  CountFromType=Initial value  CountFrom=0  CountResetPort=on  CountLoadPort=off  CountEnbPort=on  CountDirPort=off  CountDataType=Unsigned  CountWordLen=4  CountFracLen=0  CountSampTime=1
  HDL Counter3 : hdlsllib/HDL Operations/HDL Counter  CountType=Free running  CountInit=0  CountStep=1  CountMax=1  CountFromType=Initial value  CountFrom=0  CountResetPort=off  CountLoadPort=on  CountEnbPort=on  CountDirPort=off  CountDataType=Unsigned  CountWordLen=5  CountFracLen=0  CountSampTime=1
  HDL Counter4 : hdlsllib/HDL Operations/HDL Counter  CountType=Free running  CountInit=0  CountStep=1  CountMax=1  CountFromType=Initial value  CountFrom=0  CountResetPort=on  CountLoadPort=off  CountEnbPort=on  CountDirPort=off  CountDataType=Unsigned  CountWordLen=8  CountFracLen=0  CountSampTime=1
  Index Vector : MultiPortSwitch  DataPortOrder=Zero-based contiguous  Inputs=8  zeroidx=on
  Logical Operator{,3,7,9,12..20,33,36,38..46} (24 alike) : Logic  AllPortsSameDT=off  OutDataTypeStr=boolean
  Logical Operator{1,10..11,34..35} (5 alike) : Logic  Operator=OR  AllPortsSameDT=off  OutDataTypeStr=boolean
  Logical Operator{2,5..6,32} (4 alike) : Logic  Operator=XOR  AllPortsSameDT=off  OutDataTypeStr=boolean
  Logical Operator22 : Logic  Inputs=3  AllPortsSameDT=off  OutDataTypeStr=boolean
  Logical Operator25 : Logic  Inputs=3  AllPortsSameDT=off  OutDataTypeStr=boolean
  Logical Operator37 : Logic  Operator=NOT  AllPortsSameDT=off  OutDataTypeStr=boolean
  Logical Operator4 : Logic  Operator=NOT  AllPortsSameDT=off  OutDataTypeStr=boolean
  Logical Operator47 : Logic  Operator=NOT  Inputs=3  AllPortsSameDT=off  OutDataTypeStr=boolean
  Logical Operator8 : Logic  Operator=OR  Inputs=3  AllPortsSameDT=off  OutDataTypeStr=boolean
  SA12 : simulink/Additional Math & Discrete/Additional Discrete/Unit Delay Enabled  vinit=0  tsamp=-1
  Switch{1..14} (14 alike) : Switch  Criteria=u2 ~= 0
  Unit Delay Enabled Resettable : Subsystem
  Unit Delay Enabled Resettable1 : Subsystem
  Unit Delay Enabled Resettable11 : Subsystem
  Unit Delay Enabled Resettable12 : Subsystem
  Unit Delay Enabled Resettable13 : Subsystem
  Unit Delay Enabled Resettable14 : Subsystem
  Unit Delay Enabled Resettable15 : Subsystem
  Unit Delay Enabled Resettable16 : Subsystem
  Unit Delay Enabled Resettable17 : Subsystem
  Unit Delay Enabled Resettable18 : Subsystem
  Unit Delay Enabled Resettable19 : Subsystem
  Unit Delay Enabled Resettable2 : Subsystem
  Unit Delay Enabled Resettable3 : Subsystem
  Unit Delay Enabled Resettable4 : Subsystem
  Unit Delay Enabled Resettable5 : Subsystem
  Unit Delay Enabled Resettable6 : Subsystem
  Unit Delay Enabled Resettable7 : Subsystem
  Unit Delay Enabled Resettable8 : Subsystem
  Unit Delay Enabled Resettable9 : Subsystem
  signal_edg : Subsystem
  AddrOUT : Outport  OutDataTypeStr=uint8
  STATUS : Outport  Port=2  OutDataTypeStr=uint32
  Strob : Outport  Port=3  OutDataTypeStr=boolean
  wires:
  RST/1 -> Bit Slice1/1
  IO/1 -> Logical Operator25/2, [data]
  STOP/1 -> Logical Operator9/2, Logical Operator5/2, Delay1/1
  adr_IN/1 -> Delay9/1, Delay7/1
  data_in/1 -> Switch12/1, Delay11/1
  Add/1 -> Data Type Conversion9/1
  Add1/1 -> Data Type Conversion10/1
  Bit Concat/1 -> Data Type Conversion/1
  Bit Concat1/1 -> Switch3/1
  Bit Slice1/1 -> Logical Operator25/1
  Bit Slice2/1 -> Compare To Constant19/1, Compare To Constant18/1
  Bit Slice3/1 -> Data Type Conversion5/1
  Bit Slice4/1 -> Compare To Constant20/1
  Bit Slice5/1 -> Data Type Conversion1/1
  Compare To Constant1/1 -> Logical Operator/1
  Compare To Constant10/1 -> Logical Operator19/1
  Compare To Constant11/1 -> Logical Operator20/1
  Compare To Constant13/1 -> Logical Operator22/1
  Compare To Constant14/1 -> Logical Operator18/1
  Compare To Constant15/1 -> Logical Operator37/1
  Compare To Constant16/1 -> Switch11/2, [Send_com]
  Compare To Constant17/1 -> Switch8/2, Logical Operator34/2, HDL Counter4/1
  Compare To Constant18/1 -> Switch7/2, HDL Counter3/1, [WE]
  Compare To Constant19/1 -> Switch9/2
  Compare To Constant2/1 -> Logical Operator7/2, Logical Operator6/2, Delay2/1
  Compare To Constant20/1 -> Data Type Conversion3/1
  Compare To Constant21/1 -> Logical Operator39/1
  Compare To Constant22/1 -> Logical Operator40/1
  Compare To Constant23/1 -> Logical Operator41/1
  Compare To Constant24/1 -> Logical Operator42/1
  Compare To Constant25/1 -> Logical Operator43/1
  Compare To Constant26/1 -> Logical Operator44/1
  Compare To Constant27/1 -> Logical Operator45/1
  Compare To Constant28/1 -> Logical Operator46/1
  Compare To Constant29/1 -> Switch12/2
  Compare To Constant3/1 -> Logical Operator12/2
  Compare To Constant30/1 -> Unit Delay Enabled Resettable17/2(Enb), Unit Delay Enabled Resettable17/1(data_in)
  Compare To Constant31/1 -> Logical Operator38/1
  Compare To Constant32/1 -> Unit Delay Enabled Resettable17/3(Reset)
  Compare To Constant4/1 -> Logical Operator8/1, Logical Operator/2, HDL Counter1/2
  Compare To Constant5/1 -> Logical Operator13/1
  Compare To Constant6/1 -> Logical Operator14/1
  Compare To Constant7/1 -> Logical Operator15/1
  Compare To Constant8/1 -> Logical Operator16/1
  Compare To Constant9/1 -> Logical Operator17/1
  Constant/1 -> Switch1/3
  Constant1/1 -> Switch2/3
  Constant10/1 -> Switch8/1
  Constant11/1 -> Switch5/3
  Constant12/1 -> Switch3/3
  Constant13/1 -> Switch12/3
  Constant14/1 -> Switch11/3
  Constant15/1 -> Switch14/3
  Constant16/1 -> Switch13/3
  Constant17/1 -> Switch13/1
  Constant18/1 -> Switch14/1
  Constant2/1 -> Switch2/1
  Constant3/1 -> Switch7/3
  Constant4/1 -> Switch10/1
  Constant5/1 -> Switch4/3
  Constant6/1 -> Switch5/1
  Constant7/1 -> Switch9/3
  Constant8/1 -> Switch10/3
  Constant9/1 -> Logical Operator22/3
  Data Type Conversion/1 -> Switch1/1
  Data Type Conversion1/1 -> [addRd]
  Data Type Conversion10/1 -> Delay8/1
  Data Type Conversion2/1 -> [Num_Count]
  Data Type Conversion3/1 -> [RD]
  Data Type Conversion4/1 -> Add/1
  Data Type Conversion5/1 -> Switch7/1
  Data Type Conversion6/1 -> [VAL_COUNT]
  Data Type Conversion7/1 -> Bit Concat1/3
  Data Type Conversion8/1 -> Index Vector/1
  Data Type Conversion9/1 -> Delay6/1
  Delay/1 -> Logical Operator2/1
  Delay1/1 -> Logical Operator5/1
  Delay11/1 -> Switch11/1
  Delay2/1 -> Logical Operator6/1
  Delay3/1 -> [Number_bit]
  Delay4/1 -> Logical Operator32/1
  Delay5/1 -> Unit Delay Enabled Resettable9/3(Reset), Unit Delay Enabled Resettable8/3(Reset), Unit Delay Enabled Resettable7/3(Reset), Unit Delay Enabled Resettable6/3(Reset), Unit Delay Enabled Resettable5/3(Reset), Unit Delay Enabled Resettable4/3(Reset), Unit Delay Enabled Resettable3/3(Reset), Unit Delay Enabled Resettable2/3(Reset), Unit Delay Enabled Resettable1/3(Reset)
  Delay6/1 -> STATUS/1
  Delay7/1 -> Compare To Constant16/1
  Delay8/1 -> AddrOUT/1
  Delay9/1 -> Compare To Constant29/1
  [bait_done] -> Logical Operator1/1
  [data] -> Unit Delay Enabled Resettable9/1(data_in), Unit Delay Enabled Resettable8/1(data_in), Unit Delay Enabled Resettable7/1(data_in), Unit Delay Enabled Resettable6/1(data_in), Unit Delay Enabled Resettable5/1(data_in), Unit Delay Enabled Resettable4/1(data_in), Unit Delay Enabled Resettable3/1(data_in), Unit Delay Enabled Resettable2/1(data_in), Unit Delay Enabled Resettable1/1(data_in)
  [data] -> Compare To Constant31/1
  [detect_error] -> Logical Operator47/1
  [Mes_res] -> HDL Counter/2
  [bait_done] -> Logical Operator22/2
  [Error_bait] -> Logical Operator33/2, Logical Operator32/2, Delay4/1
  [Error_bait] -> Switch6/2, Switch5/2, Switch4/2, Logical Operator36/1
  [bait] -> Switch4/1
  [Num_Count] -> Bit Concat1/2
  [bait_done] -> Delay5/1
  [Read_Byte] -> Bit Concat1/1
  [RST] -> Unit Delay Enabled Resettable19/3(Reset), Unit Delay Enabled Resettable18/3(Reset), Unit Delay Enabled Resettable16/3(Reset), Unit Delay Enabled Resettable15/3(Reset), Unit Delay Enabled Resettable14/3(Reset), Unit Delay Enabled Resettable13/3(Reset), Unit Delay Enabled Resettable12/3(Reset), Unit Delay Enabled Resettable11/3(Reset)
  [VAL_COUNT] -> HDL Counter3/2
  [RD] -> Switch10/2, Logical Operator35/2
  [bait_done] -> Logical Operator10/1
  [addRd] -> Switch6/3
  [data_detect_error] -> Add/2
  [addr_detect_error] -> Add1/2
  [bait_done] -> Logical Operator11/1
  [bait_done] -> Logical Operator8/2
  [RST] -> Logical Operator8/3
  [RST] -> Logical Operator10/2
  [RST] -> Logical Operator11/2
  [Get_val] -> Logical Operator20/2, Logical Operator19/2, Logical Operator18/2, Logical Operator17/2, Logical Operator16/2, Logical Operator15/2, Logical Operator14/2, Logical Operator13/2, Logical Operator12/1
  [Number_bit] -> Compare To Constant9/1, Compare To Constant8/1, Compare To Constant7/1, Compare To Constant6/1, Compare To Constant5/1, Compare To Constant3/1, Compare To Constant14/1, Compare To Constant11/1, Compare To Constant10/1
  HDL Counter/1 -> Compare To Constant4/1
  HDL Counter1/1 -> Compare To Constant1/1
  HDL Counter2/1 -> Compare To Constant2/1, Delay3/1
  HDL Counter3/1 -> Switch6/1, Data Type Conversion2/1, Compare To Constant15/1
  HDL Counter4/1 -> Compare To Constant17/1
  Index Vector/1 -> [Read_Byte]
  Logical Operator/1 -> Switch8/3, Logical Operator34/1, HDL Counter2/2, [Get_val]
  Logical Operator1/1 -> Unit Delay Enabled Resettable/3(Reset)
  Logical Operator10/1 -> HDL Counter1/1
  Logical Operator11/1 -> HDL Counter2/1
  Logical Operator12/1 -> Unit Delay Enabled Resettable1/2(Enb)
  Logical Operator13/1 -> Unit Delay Enabled Resettable2/2(Enb)
  Logical Operator14/1 -> Unit Delay Enabled Resettable3/2(Enb)
  Logical Operator15/1 -> Unit Delay Enabled Resettable4/2(Enb)
  Logical Operator16/1 -> Unit Delay Enabled Resettable5/2(Enb)
  Logical Operator17/1 -> Unit Delay Enabled Resettable6/2(Enb)
  Logical Operator18/1 -> Unit Delay Enabled Resettable7/2(Enb)
  Logical Operator19/1 -> Unit Delay Enabled Resettable8/2(Enb)
  Logical Operator2/1 -> Logical Operator3/1
  Logical Operator20/1 -> Unit Delay Enabled Resettable9/2(Enb)
  Logical Operator22/1 -> Switch1/2, [Error_bait]
  Logical Operator25/1 -> Logical Operator4/1, Logical Operator2/2, Delay/1
  Logical Operator3/1 -> Unit Delay Enabled Resettable/2(Enb), Unit Delay Enabled Resettable/1(data_in)
  Logical Operator32/1 -> Logical Operator33/1
  Logical Operator33/1 -> Logical Operator35/1
  Logical Operator34/1 -> SA12/2
  Logical Operator35/1 -> Switch3/2, Switch2/2
  Logical Operator36/1 -> HDL Counter3/3
  Logical Operator37/1 -> Logical Operator36/2
  Logical Operator38/1 -> signal_edg/1(In1)
  Logical Operator39/1 -> Unit Delay Enabled Resettable11/2(Enb)
  Logical Operator4/1 -> Logical Operator3/2
  Logical Operator40/1 -> Unit Delay Enabled Resettable12/2(Enb)
  Logical Operator41/1 -> Unit Delay Enabled Resettable13/2(Enb)
  Logical Operator42/1 -> Unit Delay Enabled Resettable14/2(Enb)
  Logical Operator43/1 -> Unit Delay Enabled Resettable15/2(Enb)
  Logical Operator44/1 -> Unit Delay Enabled Resettable16/2(Enb)
  Logical Operator45/1 -> Unit Delay Enabled Resettable18/2(Enb)
  Logical Operator46/1 -> Unit Delay Enabled Resettable19/2(Enb)
  Logical Operator47/1 -> Logical Operator25/3
  Logical Operator5/1 -> Logical Operator9/1
  Logical Operator6/1 -> Logical Operator7/1
  Logical Operator7/1 -> [bait_done]
  Logical Operator8/1 -> HDL Counter/1
  Logical Operator9/1 -> Logical Operator1/2, [RST]
  SA12/1 -> HDL Counter4/2, Strob/1
  Switch1/1 -> [bait]
  Switch10/1 -> Data Type Conversion7/1
  Switch11/1 -> Switch9/1, Bit Slice3/1, Bit Slice2/1
  Switch12/1 -> Compare To Constant32/1, Compare To Constant30/1
  Switch13/1 -> [addr_detect_error]
  Switch14/1 -> [data_detect_error]
  Switch2/1 -> Add1/1
  Switch3/1 -> Data Type Conversion4/1
  Switch4/1 -> Unit Delay Enabled Resettable19/1(data_in), Unit Delay Enabled Resettable18/1(data_in), Unit Delay Enabled Resettable16/1(data_in), Unit Delay Enabled Resettable15/1(data_in), Unit Delay Enabled Resettable14/1(data_in), Unit Delay Enabled Resettable13/1(data_in), Unit Delay Enabled Resettable12/1(data_in), Unit Delay Enabled Resettable11/1(data_in)
  Switch5/1 -> Logical Operator46/2, Logical Operator45/2, Logical Operator44/2, Logical Operator43/2, Logical Operator42/2, Logical Operator41/2, Logical Operator40/2, Logical Operator39/2
  Switch6/1 -> Data Type Conversion8/1, Compare To Constant28/1, Compare To Constant27/1, Compare To Constant26/1, Compare To Constant25/1, Compare To Constant24/1, Compare To Constant23/1, Compare To Constant22/1, Compare To Constant21/1
  Switch7/1 -> Data Type Conversion6/1
  Switch8/1 -> SA12/1
  Switch9/1 -> Bit Slice5/1, Bit Slice4/1
  Unit Delay Enabled Resettable/1(data_out) -> [Mes_res]
  Unit Delay Enabled Resettable1/1(data_out) -> Compare To Constant13/1
  Unit Delay Enabled Resettable11/1(data_out) -> Index Vector/2
  Unit Delay Enabled Resettable12/1(data_out) -> Index Vector/3
  Unit Delay Enabled Resettable13/1(data_out) -> Index Vector/4
  Unit Delay Enabled Resettable14/1(data_out) -> Index Vector/5
  Unit Delay Enabled Resettable15/1(data_out) -> Index Vector/6
  Unit Delay Enabled Resettable16/1(data_out) -> Index Vector/7
  Unit Delay Enabled Resettable17/1(data_out) -> Logical Operator38/2, [detect_error]
  Unit Delay Enabled Resettable18/1(data_out) -> Index Vector/8
  Unit Delay Enabled Resettable19/1(data_out) -> Index Vector/9
  Unit Delay Enabled Resettable2/1(data_out) -> Bit Concat/1
  Unit Delay Enabled Resettable3/1(data_out) -> Bit Concat/2
  Unit Delay Enabled Resettable4/1(data_out) -> Bit Concat/3
  Unit Delay Enabled Resettable5/1(data_out) -> Bit Concat/4
  Unit Delay Enabled Resettable6/1(data_out) -> Bit Concat/5
  Unit Delay Enabled Resettable7/1(data_out) -> Bit Concat/6
  Unit Delay Enabled Resettable8/1(data_out) -> Bit Concat/7
  Unit Delay Enabled Resettable9/1(data_out) -> Bit Concat/8
  signal_edg/1(Out1) -> Switch14/2, Switch13/2

== system gm_smartCart3111/head/switch_io ==
  IO : Inport  OutDataTypeStr=boolean
  IO_IN : Inport  Port=2  OutDataTypeStr=boolean
  switch_io : Inport  Port=3  OutDataTypeStr=boolean  SampleTime=1
  Out1 : Outport  OutDataTypeStr=boolean
  wires:
  IO/1 -> Out1/1
